simulink model "arduino_serial_gps"  (R2024b)
settings: Solver=FixedStepAuto  StartTime=0.0  StopTime=50  RelTol=1e-3
libraries: arduinolib x2
settings Model: SimulationMode=external  ExtModeTrigDuration=2  ExtModeArchiveDirName=C:\Users\mmordeka\Desktop\2_6_morning  ExtModeAddSuffixToVar=on  Creator=The MathWorks, Inc.  LastModifiedBy=Nitesh
settings SolverCC: AlgebraicLoopSolver=TrustRegion  AutoInsertRateTranBlk=on
settings DataIOCC: ReturnWorkspaceOutputs=off
settings OptimizationCC: EnhancedBackFolding=on  PassReuseOutputArgsAs=Individual arguments  ZeroExternalMemoryAtStartup=off  ZeroInternalMemoryAtStartup=off  MaxStackSize=64  OptimizeBlockOrder=speed  DifferentSizesBufferReuse=on  OptimizationCustomize=off  EfficientTunableParamExpr=on
settings DebuggingCC: ParameterTunabilityLossMsg=error  UnconnectedInputMsg=warning  UnconnectedOutputMsg=warning  UnconnectedLineMsg=warning  ArithmeticOperatorsInVariantConditions=warning
settings HardwareCC: ProdBitPerPointer=32  ProdBitPerSizeT=32  ProdBitPerPtrDiffT=32  ProdLargestAtomicInteger=Long  ProdLargestAtomicFloat=Double  ProdWordSize=32  ProdHWDeviceType=ARM Compatible->ARM Cortex  UseEmbeddedCoderFeatures=off
settings ModelReferenceCC: EnableRefExpFcnMdlSchedulingChecks=on
settings SFSimCC: SimUseLocalCustomCode=off  MATLABDynamicMemAlloc=off
settings RTWCC: Description=Embedded Coder  SystemTargetFile=ert.tlc  HardwareBoard=ESP32-WROOM(Arduino Compatible)  TLCOptions="-aInlineSetEventsForThisBaseRateFcn=TLC_FALSE -aSuppressMultiTaskScheduler=TLC_FALSE  -aRateBasedStepFcn=0"  TemplateMakefile=ert_default_tmf  RTWUseLocalCustomCode=off  CustomHeaderCode=include\gps_parser.h  CustomSource=src\gps_parser.cpp  Toolchain=ESP32  BuildConfiguration=Debug  GPUComputeCapability=3.5
settings RTWCC: CustomInclude=|
  | src\
  | include\
settings CodeAppCC: ForceParamTrailComments=on  IgnoreCustomStorageClasses=off  OperatorAnnotations=on  SimulinkDataObjDesc=on  SFDataObjDesc=on  InsertBlockDesc=on
settings ERTTargetCC: SupportContinuousTime=on  SupportNonInlinedSFcns=on  SupportVariableSizeSignals=on  ExtModeTransport=3  ExtModeStaticAlloc=on  ExtModeAutomaticAllocSize=off  ExtModeStaticAllocSize=65536  ExtModeMexFile=ext_xcp  ExtModeIntrfLevel=Level2 - Open  InlinedParameterPlacement=Hierarchical

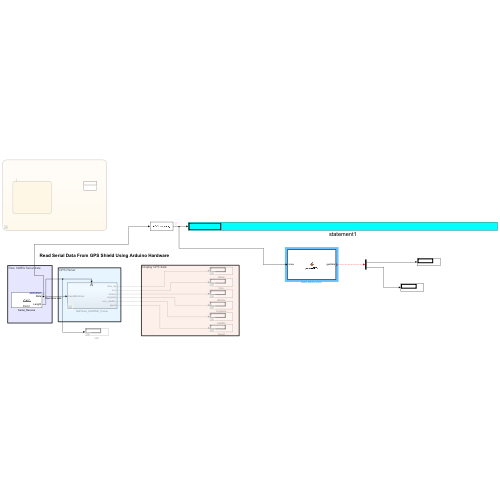
[thumbnail: Simulink's stored preview of the top-level diagram]
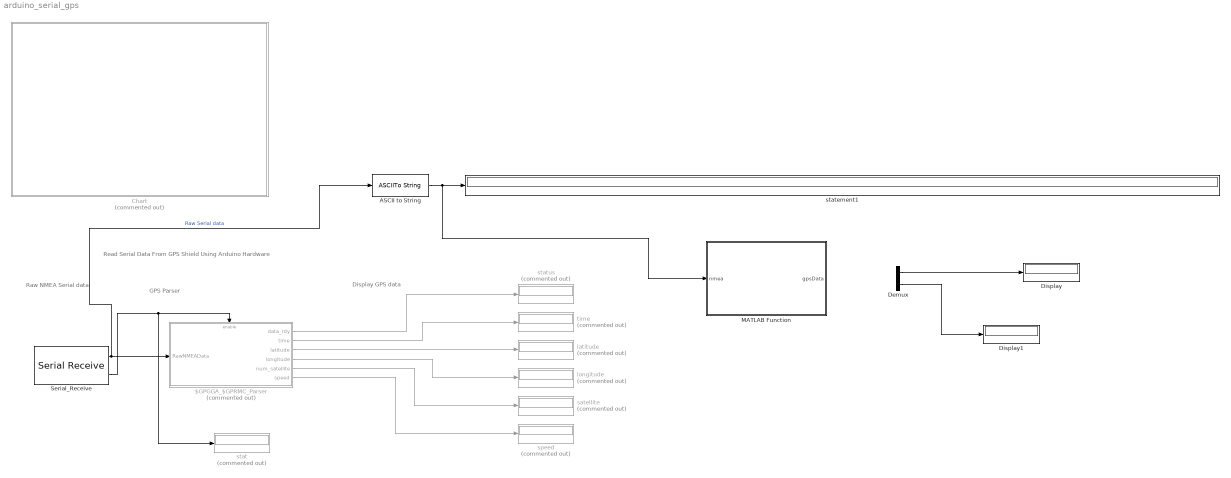
== system arduino_serial_gps ==
  note: Display GPS data
  note: GPS Parser
  note: Raw NMEA Serial data
  note: Read Serial Data From GPS Shield Using Arduino Hardware
  $GPGGA_$GPRMC_Parser : Subsystem  Commented=on  TreatAsAtomicUnit=on
  ASCII to String : ASCIIToString
  Chart : Stateflow chart  Commented=on  TreatAsAtomicUnit=on
  Demux : Demux  Outputs=2
  Display : Display
  Display1 : Display
  MATLAB Function : MATLAB Function  TreatAsAtomicUnit=on
  Serial_Receive : arduinolib/Serial Receive  portNumber=2  DataType=uint8  blockPlatform=arduino  TimeOut=0  MaxDataLength=80  isARMArch=off  DataLengthOption=Variable length  Datalength=32  Header=[36]  Terminator=[36]  SampleTime=0.05  ShowOutStatus=on
      settings: SourceProductName=Common
  latitude : Display  Commented=on
  longitude : Display  Commented=on
  satellite : Display  Commented=on
  speed : Display  Commented=on
  stat : Display  Commented=on
  statement1 : Display
  status : Display  Commented=on
  time : Display  Commented=on
  wires:
  Serial_Receive/1 -> $GPGGA_$GPRMC_Parser/1(RawNMEAData), ASCII to String/1  "Raw Serial data"
  Serial_Receive/2 -> stat/1, $GPGGA_$GPRMC_Parser/Enable
  $GPGGA_$GPRMC_Parser/3(latitude) -> latitude/1
  $GPGGA_$GPRMC_Parser/1(data_rdy) -> status/1
  $GPGGA_$GPRMC_Parser/6(speed) -> speed/1
  $GPGGA_$GPRMC_Parser/2(time) -> time/1
  $GPGGA_$GPRMC_Parser/5("num_satellite ") -> satellite/1
  $GPGGA_$GPRMC_Parser/4(longitude) -> longitude/1
  ASCII to String/1 -> MATLAB Function/1(nmea), statement1/1
  ? -> Demux/1
  Demux/1 -> Display/1
  Demux/2 -> Display1/1

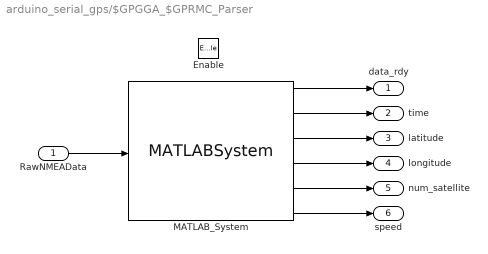
== system arduino_serial_gps/$GPGGA_$GPRMC_Parser ==
  RawNMEAData : Inport
  Enable : EnablePort  StatesWhenEnabling=reset
  MATLAB_System : MATLABSystem  System=GPSParser  TimeOpt=on  LatOpt=on  LonOpt=on  NoSatOpt=on  HdopOpt=off  AltOpt=off  MslOpt=off  SpeedOpt=on  DateOpt=off  TckAngOpt=off
      mask Type: GPSParser
      mask Display:
      | disp('GPSParser');
      | port_label('input',1,'inData');
      | port_label('output',1,'Status');
      | port_label('output',2,'Time');
      | port_label('output',3,'Latitude');
      | port_label('output',4,'Longitude');
      | port_label('output',5,'Satellite');
      | port_label('output',6,'Speed');
  data_rdy : Outport  OutputWhenDisabled=reset  InitialOutput=0  VectorParamsAs1DForOutWhenUnconnected=off
  time : Outport  Port=2  OutputWhenDisabled=reset  InitialOutput=0  VectorParamsAs1DForOutWhenUnconnected=off
  latitude : Outport  Port=3  OutputWhenDisabled=reset  InitialOutput=0  VectorParamsAs1DForOutWhenUnconnected=off
  longitude : Outport  Port=4  OutputWhenDisabled=reset  InitialOutput=0  VectorParamsAs1DForOutWhenUnconnected=off
  "num_satellite " : Outport  Port=5  OutputWhenDisabled=reset  InitialOutput=0  VectorParamsAs1DForOutWhenUnconnected=off
  speed : Outport  Port=6  OutputWhenDisabled=reset  InitialOutput=0  VectorParamsAs1DForOutWhenUnconnected=off
  wires:
  MATLAB_System/1 -> data_rdy/1
  RawNMEAData/1 -> MATLAB_System/1
  MATLAB_System/2 -> time/1
  MATLAB_System/3 -> latitude/1
  MATLAB_System/4 -> longitude/1
  MATLAB_System/5 -> "num_satellite "/1
  MATLAB_System/6 -> speed/1

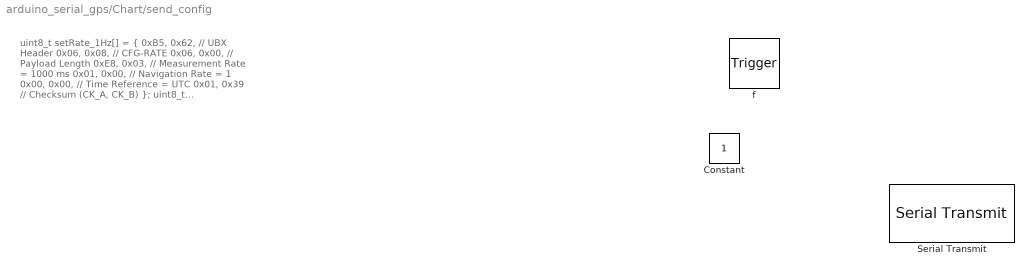
== system arduino_serial_gps/Chart/send_config ==
  note: uint8_t setRate_1Hz[] = {
      |   0xB5, 0x62,  // UBX Header
      |   0x06, 0x08,  // CFG-RATE
      |   0x06, 0x00,  // Payload Length
      |   0xE8, 0x03,  // Measurement Rate = 1000 ms
      |   0x01, 0x00,  // Navigation Rate = 1
      |   0x00, 0x00,  // Time Reference = UTC
      |   0x01, 0x39   // Checksum (CK_A, CK_B)
      | };
      |
      |
      | uint8_t setRate_2Hz[] = {
      |   0xB5, 0x62,
      |   0x06, 0x08,
      |   0x06, 0x00,
      |   0xF4, 0x01,  // Measurement Rate = 500 ms
      |   0x01, 0x00,
      |   0x00, 0x00,
      |   0x0E, 0x79   // Checksum
      | };
      |
      | uint8_t setRate_3Hz[] = {
      |   0xB5, 0x62,
      |   0x06, 0x08,
      |   0x06, 0x00,
      |   0x4D, 0x01,  // Measurement Rate = 333 ms
      |   0x01, 0x00,
      |   0x00, 0x00,
      |   0x5F, 0x52   // Checksum
      | };
      |
      | uint8_t setRate_4Hz[] = {
      |   0xB5, 0x62,
      |   0x06, 0x08,
      |   0x06, 0x00,
      |   0xFA, 0x00,  // Measurement Rate = 250 ms
      |   0x01, 0x00,
      |   0x00, 0x00,
      |   0x1F, 0x6A   // Checksum
      | };
      |
      | uint8_t setRate_5Hz[] = {
      |   0xB5, 0x62,
      |   0x06, 0x08,
      |   0x06, 0x00,
      |   0xC8, 0x00,  // Measurement Rate = 200 ms
      |   0x01, 0x00,
      |   0x00, 0x00,
      |   0xDE, 0x6A   // Checksum
      | };
  f : TriggerPort  TriggerType=function-call  VariantControl=(inherit)
      settings: CopyFcn=Stateflow.SLINSF.SimulinkMan.removeBlockPreDeleteFcn  PreDeleteFcn=Stateflow.SLINSF.SimulinkMan.unsafePredeleteFcn
  Constant : Constant
  Serial Transmit : arduinolib/Serial Transmit  portNumber=2  sendmode=write  sendformat=Decimal  floatprecision=2  header=[]  terminator=[]  blockPlatform=ARDUINO
      settings: SourceProductName=Common

== stateflow chart arduino_serial_gps/Chart ==
  state Init
  state send_config [function]
  (default) -> Init

== matlab function arduino_serial_gps/MATLAB Function ==
  data: nmea input; gpsData output <data type expression>
function gpsData = parseGPS_numeric(nmea)
% parseGPS_numeric Parses NMEA sentences from a GPS (e.g., NEO6M) and outputs
% latitude, longitude, speed, hdop, and satellites in numeric types.
%
%   gpsData = parseGPS_numeric(nmea) parses the input NMEA sentence(s) and returns
%   a structure array with the following fields:
%       latitude   - single (float32) in decimal degrees.
%       longitude  - single (float32) in decimal degrees.
%       speed      - single (float32). Speed is taken from RMC (knots) or VTG (km/h).
%       hdop       - single (float32). Horizontal dilution of precision.
%       satellites - uint8. Number of satellites.
%
%   The input 'nmea' can be a single string or a cell array of strings.
%
%   Example:
%       sentences = {
%           '$GPGGA,123519,4807.038,N,01131.000,E,1,08,0.9,545.4,M,46.9,M,,*47'
%           '$GPRMC,225446,A,4916.45,N,12311.12,W,000.5,054.7,191194,020.3,E*68'
%       };
%       data = parseGPS_numeric(sentences);
%
% Author: [Your Name]
% Date: [Date]

% Ensure input is a cell array
if ischar(nmea) || isstring(nmea)
    nmea = cellstr(nmea);
end

% Initialize output structure array.
gpsData = repmat(struct('latitude', single(NaN), 'longitude', single(NaN), ...
    'speed', single(NaN), 'hdop', single(NaN), 'satellites', uint8(0)), length(nmea), 1);

for i = 1:length(nmea)
    sentence = strtrim(nmea{i});
    if isempty(sentence)
        continue;
    end
    
    % Remove leading '$' if present
    if sentence(1) == '$'
        sentence = sentence(2:end);
    end
    
    % Remove checksum (if present) by splitting at '*'
    parts = split(sentence, '*');
    core = parts{1}; % everything before the checksum
    
    % Split the core sentence by commas
    tokens = split(core, ',');
    if isempty(tokens)
        continue;
    end
    
    % The first token contains the talker and sentence type (e.g., 'GPGGA')
    idStr = tokens{1};
    if length(idStr) >= 5
        sentenceType = idStr(3:end);
    else
        sentenceType = idStr;
    end
    
    % Use a temporary structure to hold parsed numeric fields.
    entry.latitude   = single(NaN);
    entry.longitude  = single(NaN);
    entry.speed      = single(NaN);
    entry.hdop       = single(NaN);
    entry.satellites = uint8(0);
    
    switch sentenceType
        case 'GGA'
            % Expected format:
            % Time, Latitude, N/S, Longitude, E/W, FixQuality, NumSatellites, HDOP, Altitude, ...
            if numel(tokens) >= 9
                % Convert latitude and longitude (ddmm.mmmm and dddmm.mmmm format)
                latStr = tokens{2};
                ns     = tokens{3};
                lonStr = tokens{5};
                ew     = tokens{6};
                latVal = convertNMEALatLon(latStr, ns);
                lonVal = convertNMEALatLon(lonStr, ew);
                
                entry.latitude  = single(latVal);
                entry.longitude = single(lonVal);
                entry.hdop      = single(str2double(tokens{9}));
                entry.satellites = uint8(str2double(tokens{8}));
            end
            
        case 'RMC'
            % Expected format:
            % Time, Status, Latitude, N/S, Longitude, E/W, Speed (knots), Course, Date, ...
            if numel(tokens) >= 8
                latStr = tokens{4};
                ns     = tokens{5};
                lonStr = tokens{6};
                ew     = tokens{7};
                latVal = convertNMEALatLon(latStr, ns);
                lonVal = convertNMEALatLon(lonStr, ew);
                
                entry.latitude  = single(latVal);
                entry.longitude = single(lonVal);
                entry.speed     = single(str2double(tokens{8})); % speed in knots
            end
            
        case 'VTG'
            % Expected format:
            % Track true, 'T', Track magnetic, 'M', Speed (knots), 'N', Speed (km/h), 'K'
            if numel(tokens) >= 9
                entry.speed = single(str2double(tokens{8})); % speed in km/h
            end
            
        otherwise
            % For sentences that do not include these fields, do nothing.
    end
    
    gpsData(i) = entry;
end

end

function dec = convertNMEALatLon(str, direction)
% convertNMEALatLon Converts a NMEA latitude/longitude string to decimal degrees.
%   For latitude, the format is ddmm.mmmm and for longitude, dddmm.mmmm.
%
%   str: a string representing the coordinate (e.g., '4807.038' or '01131.000')
%   direction: 'N', 'S', 'E', or 'W'

    if isempty(str) || any(isnan(str2double(str)))
        dec = NaN;
        return;
    end
    
    % Use the direction to decide whether degrees are 2 or 3 digits.
    if direction == 'N' || direction == 'S'
        % Latitude: first 2 digits are degrees.
        deg = str2double(str(1:2));
        min = str2double(str(3:end));
    elseif direction == 'E' || direction == 'W'
        % Longitude: first 3 digits are degrees.
        deg = str2double(str(1:3));
        min = str2double(str(4:end));
    else
        dec = NaN;
        return;
    end
    
    dec = deg + min/60;
    
    % South or West are negative.
    if direction == 'S' || direction == 'W'
        dec = -dec;
    end
end
